simulink model "s"  (R2023a)
settings: Solver=VariableStepAuto  StartTime=0.0  StopTime=10  RelTol=1e-3
InitFcn:
  | Rm=3.15;
  | Lm=0.0015;
  | K=1.028;
  | k=1.028;
  | fm=0.16805;
  | A2=0.0033153;
  | A1=0.045721;
  | L01=0.2625;
  | m2=0.24355;
  | A1tilde=A1+A2+m2*L01*L01;
  | A2tilde=A1tilde-A2;
  | f=0.070633;
  | lg1=0.16655703376925832;
  | m1=0.66984;
  | g=9.8;
  | Ceq=L01*m2*g+lg1*m1*g;
  | CONS4=(A2*A1tilde-A2*A2tilde)*Lm/K;
  | CONS3=(A2*(A1tilde-A2tilde)*(Rm/K)+(Lm/K)*(f*A2+A1tilde*fm));
  | CONS2=((Rm/K)*(f*A2+A1tilde*fm)+(Lm/K)*((f*fm-Ceq*A2)+K*f));
  | CONS1=((Rm/K)*(f*fm-Ceq*A2)-(Lm/k *Ceq*fm)+K*f);
  | CONS0=-Rm/K * Ceq * fm-K*Ceq;
settings Model: Creator=mimom  LastModifiedBy=mimom

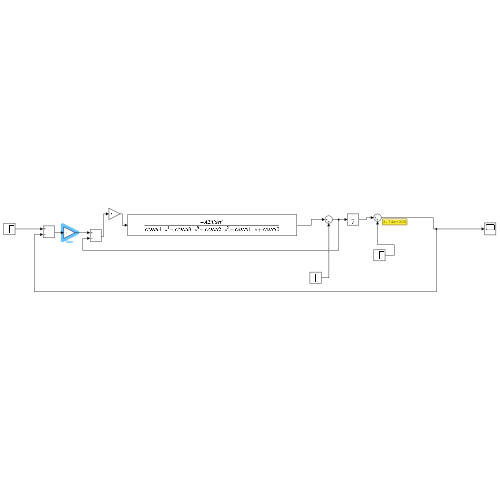
[thumbnail: Simulink's stored preview of the top-level diagram]
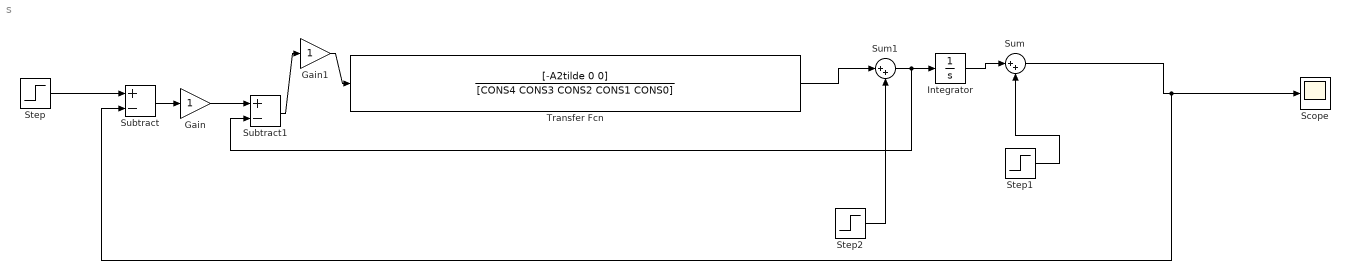
== system s ==
  Gain : Gain
  Gain1 : Gain
  Integrator : Integrator
  Scope : Scope
  Step : Step  Time=30  After=0  SampleTime=0
  Step1 : Step  Time=0.1  After=0  SampleTime=0
  Step2 : Step  Time=0.1  Before=1  After=0  SampleTime=0
  Subtract : Sum  Inputs=+-
  Subtract1 : Sum  Inputs=+-
  Sum : Sum  Inputs=|++
  Sum1 : Sum  Inputs=|++
  Transfer Fcn : TransferFcn  Numerator=[-A2tilde 0 0]  Denominator=[CONS4 CONS3 CONS2 CONS1 CONS0]
  wires:
  Step/1 -> Subtract/1
  Subtract/1 -> Gain/1
  Step1/1 -> Sum/2
  Sum/1 -> Subtract/2, Scope/1
  Integrator/1 -> Sum/1
  Gain/1 -> Subtract1/1
  Subtract1/1 -> Gain1/1
  Gain1/1 -> Transfer Fcn/1
  Sum1/1 -> Subtract1/2, Integrator/1
  Transfer Fcn/1 -> Sum1/1
  Step2/1 -> Sum1/2
